simulink model "EDS_Simulink_Model_02"  (R2022a)
settings: Solver=VariableStepAuto  StartTime=0.0  StopTime=stop_time  MaxStep=1e-5  RelTol=1e-3
values from neighbouring files (symbols this model uses):
  a = a/180*pi    [EDS_Script_Model_01.m]    (also in EDS_Script_Model_02.m)
  accel = wheel_radps/accel_time    [EDS_Script_Model_01.m]    (also in EDS_Script_Model_02.m)
  accel_time = 5.33    [EDS_Script_Model_01.m]    (also in EDS_Script_Model_02.m)
  Cx = 0.25    [EDS_Script_Model_01.m]    (also in EDS_Script_Model_02.m)
  d = 1.5    [EDS_Script_Model_01.m]    (also in EDS_Script_Model_02.m)
  density = 1.3    [EDS_Script_Model_01.m]    (also in EDS_Script_Model_02.m)
  F = 4e-04    (= 0.0004)    [EDS_Script_Model_02.m]
  Filter_coefficient = 100/50    (= 2)    [EDS_Script_Model_02.m]
  fr = 0.01    [EDS_Script_Model_01.m]    (also in EDS_Script_Model_02.m)
  g = 9.81    [EDS_Script_Model_01.m]    (also in EDS_Script_Model_02.m)
  i_gear = 7.2    [EDS_Script_Model_01.m]    (also in EDS_Script_Model_02.m = 1)
  J = 0.07/4    (= 0.0175)    [EDS_Script_Model_02.m]
  K_tor_all_1 = 1/2    (= 0.5)    [EDS_Script_Model_01.m]    (also in EDS_Script_Model_02.m)
  K_tor_all_2 = 1/2    (= 0.5)    [EDS_Script_Model_01.m]    (also in EDS_Script_Model_02.m)
  Kd_w = 0.5/8    (= 0.0625)    [EDS_Script_Model_02.m]
  Ki_id = 0.2/14    (= 0.0142857142857)    [EDS_Script_Model_02.m]
  Ki_iq = 10/14    (= 0.714285714286)    [EDS_Script_Model_02.m]
  Ki_w = 2/0.024    (= 83.3333333333)    [EDS_Script_Model_02.m]
  Kp_id = 5/12    (= 0.416666666667)    [EDS_Script_Model_02.m]
  Kp_iq = 30/12    (= 2.5)    [EDS_Script_Model_02.m]
  Kp_w = 55/0.024    (= 2291.66666667)    [EDS_Script_Model_02.m]
  L = 2.5    [EDS_Script_Model_01.m]    (also in EDS_Script_Model_02.m)
  M = 1200    [EDS_Script_Model_01.m]    (also in EDS_Script_Model_02.m)
  n_eff_gear = 0.98    [EDS_Script_Model_01.m]    (also in EDS_Script_Model_02.m = 1)
  p = 4    [EDS_Script_Model_02.m]
  Rs = 4.47-1.47-0.40    (= 2.6)    [EDS_Script_Model_02.m]
  Rw = 0.26    [EDS_Script_Model_01.m]    (also in EDS_Script_Model_02.m)
  S = 1.9    [EDS_Script_Model_01.m]    (also in EDS_Script_Model_02.m)
  Satur_max_PI_id = Vdc_1*sqrt(1/3)    [EDS_Script_Model_02.m]
  Satur_max_PI_iq = Vdc_1*sqrt(1/3)    [EDS_Script_Model_02.m]
  Satur_max_PI_w = 40+30    (= 70)    [EDS_Script_Model_02.m]
  Satur_min_PI_id = -Vdc_1*sqrt(1/3)    [EDS_Script_Model_02.m]
  Satur_min_PI_iq = -Vdc_1*sqrt(1/3)    [EDS_Script_Model_02.m]
  Satur_min_PI_w = -40-30    (= -70)    [EDS_Script_Model_02.m]
  steering_angle_1 = steering_angle_1_m(ii)    [EDS_Script_Model_01.m]    (also in EDS_Script_Model_02.m)
  steering_angle_2 = steering_angle_2_m(ii)    [EDS_Script_Model_01.m]    (also in EDS_Script_Model_02.m)
  steering_angle_3 = steering_angle_3_m(ii)    [EDS_Script_Model_01.m]    (also in EDS_Script_Model_02.m)
  steering_angle_4 = steering_angle_4_m(ii)    [EDS_Script_Model_01.m]    (also in EDS_Script_Model_02.m)
  steering_angle_initial = steering_angle_initial_m(ii)    [EDS_Script_Model_01.m]    (also in EDS_Script_Model_02.m)
  Tf = 0    [EDS_Script_Model_02.m]
  time_steering_angle_1 = 8    [EDS_Script_Model_01.m]    (also in EDS_Script_Model_02.m)
  time_steering_angle_2 = 10    [EDS_Script_Model_01.m]    (also in EDS_Script_Model_02.m)
  time_steering_angle_3 = 14    [EDS_Script_Model_01.m]    (also in EDS_Script_Model_02.m)
  time_steering_angle_4 = 18    [EDS_Script_Model_01.m]    (also in EDS_Script_Model_02.m)
  Vdc_1 = 500    [EDS_Script_Model_02.m]
  Vdc_2 = 500    [EDS_Script_Model_02.m]
  Vf = 0    [EDS_Script_Model_02.m]
  Vfd = 0    [EDS_Script_Model_02.m]
undefined symbols (not defined in the file or in its folder): time_w_ref_1, time_w_ref_2, w_ref_1, w_ref_2, w_ref_initial
libraries: slpidlib x6, spsPermanentMagnetSynchronousMachineLib x2, spsThreePhaseVIMeasurementLib x2, spsUniversalBridgeLib x2, spsDCVoltageSourceLib x2, spsVoltageMeasurementLib x2, spspowerguiLib x1
(part 2 of 2)

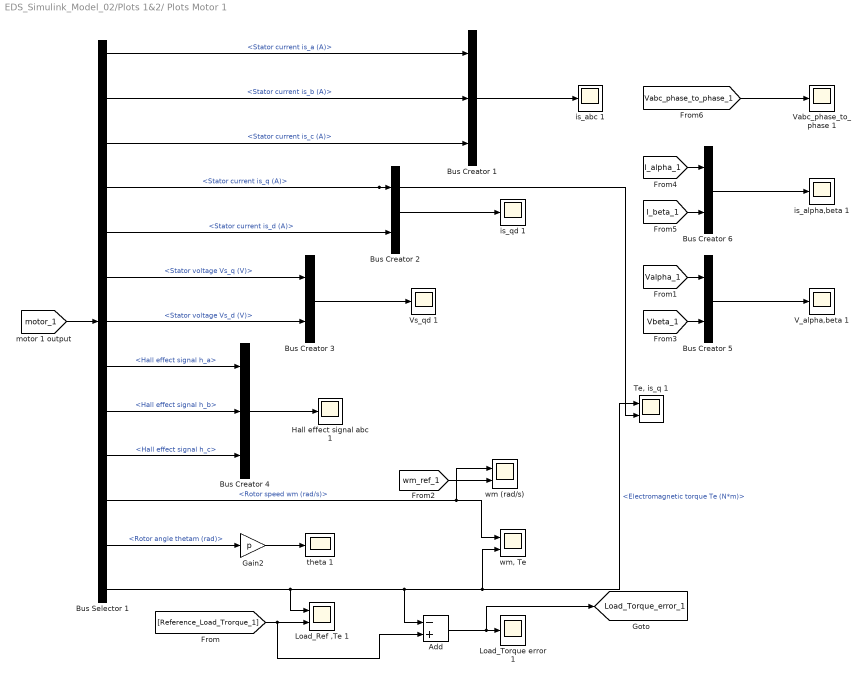
== system EDS_Simulink_Model_02/Plots 1&2/ Plots Motor 1 ==
  Add : Sum  Inputs=-+
  Bus Creator 1 : BusCreator  Inputs=3
  Bus Creator {2..3,5..6} (4 alike) : BusCreator  Inputs=2
  Bus Creator 4 : BusCreator  Inputs=3
  Bus Selector 1 : BusSelector  OutputSignals=Stator current is_a (A),Stator current is_b (A),Stator current is_c (A),Stator current is_q (A),Stator current is_d (A),Stator voltage Vs_q (V),Stator voltage Vs_d (V),Hall effect signal h_a,Hall effect signal h_b,Hall effect signal h_c,Rotor speed wm (rad/s),Rotor angle thetam (rad),Electromagnetic torque Te (N*m)
  Gain2 : Gain  Gain=p
  Hall effect signal abc 1 : Scope
  Load_Ref ,Te 1 : Scope  NumInputPorts=2
  Load_Torque error 1 : Scope
  "Te, is_q 1" : Scope  NumInputPorts=2
  V_alpha,beta 1 : Scope
  Vabc_phase_to_phase 1 : Scope
  Vs_qd 1 : Scope
  is_abc 1 : Scope
  is_alpha,beta 1 : Scope
  is_qd 1 : Scope
  theta 1 : Scope
  wm (rad/s) : Scope  NumInputPorts=2
  "wm, Te" : Scope  NumInputPorts=2
  tag scope: Load_Torque_error_1=global
  wires:
  Bus Creator 2/1 -> is_qd 1/1
  Bus Creator 3/1 -> Vs_qd 1/1
  Bus Creator 4/1 -> Hall effect signal abc 1/1
  Bus Selector 1/7 -> Bus Creator 3/2  "<Stator voltage Vs_d (V)>"
  [Vabc_phase_to_phase_1] -> Vabc_phase_to_phase 1/1
  Bus Selector 1/5 -> Bus Creator 2/2  "<Stator current is_d (A)>"
  Bus Selector 1/3 -> Bus Creator 1/3  "<Stator current is_c (A)>"
  Bus Selector 1/2 -> Bus Creator 1/2  "<Stator current is_b (A)>"
  [Valpha_1] -> Bus Creator 5/1
  [Reference_Load_Trorque_1] -> Add/2, Load_Ref ,Te 1/2
  Bus Selector 1/13 -> "Te, is_q 1"/1, "wm, Te"/2, Add/1, Load_Ref ,Te 1/1  "<Electromagnetic torque Te (N*m)>"
  Bus Selector 1/11 -> wm (rad/s)/1, "wm, Te"/1  "<Rotor speed wm (rad/s)>"
  Bus Selector 1/12 -> Gain2/1  "<Rotor angle thetam (rad)>"
  Bus Creator 5/1 -> V_alpha,beta 1/1
  Bus Selector 1/4 -> "Te, is_q 1"/2, Bus Creator 2/1  "<Stator current is_q (A)>"
  [motor_1] -> Bus Selector 1/1
  Bus Selector 1/10 -> Bus Creator 4/3  "<Hall effect signal h_c>"
  Bus Creator 1/1 -> is_abc 1/1
  Bus Selector 1/6 -> Bus Creator 3/1  "<Stator voltage Vs_q (V)>"
  Bus Selector 1/9 -> Bus Creator 4/2  "<Hall effect signal h_b>"
  [Vbeta_1] -> Bus Creator 5/2
  Bus Selector 1/1 -> Bus Creator 1/1  "<Stator current is_a (A)>"
  [I_alpha_1] -> Bus Creator 6/1
  Bus Selector 1/8 -> Bus Creator 4/1  "<Hall effect signal h_a>"
  [I_beta_1] -> Bus Creator 6/2
  Gain2/1 -> theta 1/1
  Bus Creator 6/1 -> is_alpha,beta 1/1
  Add/1 -> [Load_Torque_error_1], Load_Torque error 1/1
  [wm_ref_1] -> wm (rad/s)/2

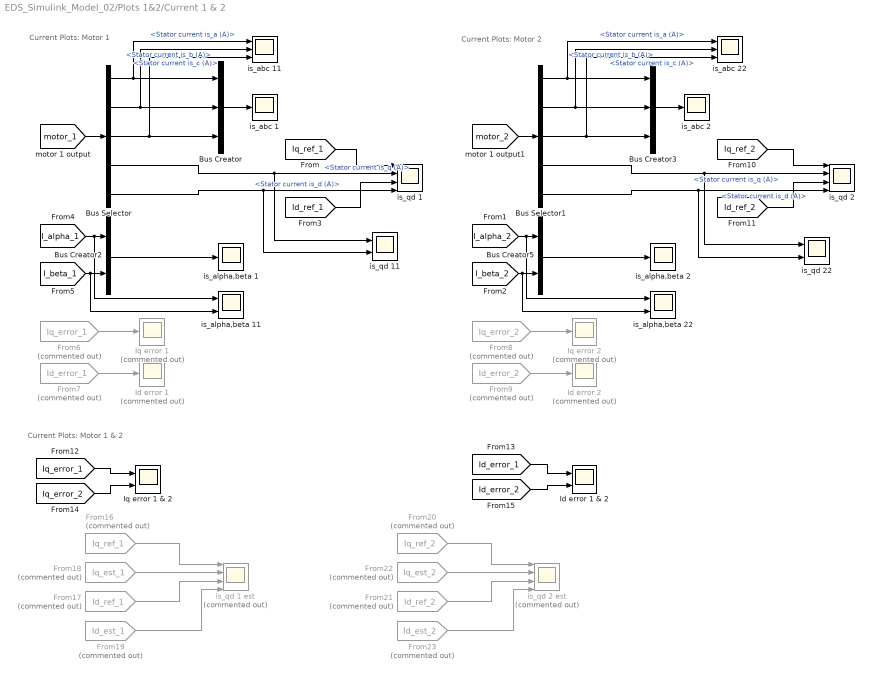
== system EDS_Simulink_Model_02/Plots 1&2/Current 1 & 2 ==
  note: Current Plots: Motor 1 & 2
  note: Current Plots: Motor 1
  note: Current Plots: Motor 2
  Bus Creator : BusCreator  Inputs=3
  Bus Creator2 : BusCreator  Inputs=2
  Bus Creator3 : BusCreator  Inputs=3
  Bus Creator5 : BusCreator  Inputs=2
  Bus Selector : BusSelector  OutputSignals=Stator current is_a (A),Stator current is_b (A),Stator current is_c (A),Stator current is_q (A),Stator current is_d (A)
  Bus Selector1 : BusSelector  OutputSignals=Stator current is_a (A),Stator current is_b (A),Stator current is_c (A),Stator current is_q (A),Stator current is_d (A)
  From16 : From  Commented=on  GotoTag=Iq_ref_1  TagVisibility=global
  From17 : From  Commented=on  GotoTag=Id_ref_1  TagVisibility=global
  From18 : From  Commented=on  GotoTag=Iq_est_1  TagVisibility=global
  From19 : From  Commented=on  GotoTag=Id_est_1  TagVisibility=global
  From20 : From  Commented=on  GotoTag=Iq_ref_2  TagVisibility=global
  From21 : From  Commented=on  GotoTag=Id_ref_2  TagVisibility=global
  From22 : From  Commented=on  GotoTag=Iq_est_2  TagVisibility=global
  From23 : From  Commented=on  GotoTag=Id_est_2  TagVisibility=global
  From6 : From  Commented=on  GotoTag=Iq_error_1  TagVisibility=global
  From7 : From  Commented=on  GotoTag=Id_error_1  TagVisibility=global
  From8 : From  Commented=on  GotoTag=Iq_error_2  TagVisibility=global
  From9 : From  Commented=on  GotoTag=Id_error_2  TagVisibility=global
  Id error 1 : Scope  Commented=on
  Id error 1 & 2 : Scope  NumInputPorts=2
  Id error 2 : Scope  Commented=on
  Iq error 1 : Scope  Commented=on
  Iq error 1 & 2 : Scope  NumInputPorts=2
  Iq error 2 : Scope  Commented=on
  is_abc 1 : Scope
  is_abc 11 : Scope  NumInputPorts=3
  is_abc 2 : Scope
  is_abc 22 : Scope  NumInputPorts=3
  is_alpha,beta 1 : Scope
  is_alpha,beta 11 : Scope  NumInputPorts=2
  is_alpha,beta 2 : Scope
  is_alpha,beta 22 : Scope  NumInputPorts=2
  is_qd 1 : Scope  NumInputPorts=4
  is_qd 1 est : Scope  Commented=on  NumInputPorts=4
  is_qd 11 : Scope  NumInputPorts=2
  is_qd 2 : Scope  NumInputPorts=4
  is_qd 2 est : Scope  Commented=on  NumInputPorts=4
  is_qd 22 : Scope  NumInputPorts=2
  wires:
  From9/1 -> Id error 2/1
  From8/1 -> Iq error 2/1
  [Id_ref_2] -> is_qd 2/3
  [I_alpha_2] -> is_alpha,beta 22/1, Bus Creator5/1
  Bus Selector1/3 -> is_abc 22/3, Bus Creator3/3  "<Stator current is_c (A)>"
  Bus Creator3/1 -> is_abc 2/1
  Bus Creator5/1 -> is_alpha,beta 2/1
  [Iq_ref_2] -> is_qd 2/1
  [motor_2] -> Bus Selector1/1
  From7/1 -> Id error 1/1
  Bus Selector/2 -> is_abc 11/2, Bus Creator/2  "<Stator current is_b (A)>"
  Bus Creator2/1 -> is_alpha,beta 1/1
  Bus Selector/3 -> Bus Creator/3, is_abc 11/3  "<Stator current is_c (A)>"
  From6/1 -> Iq error 1/1
  [Iq_ref_1] -> is_qd 1/1
  [Id_ref_1] -> is_qd 1/3
  Bus Selector/5 -> is_qd 11/2, is_qd 1/4  "<Stator current is_d (A)>"
  Bus Creator/1 -> is_abc 1/1
  [I_alpha_1] -> is_alpha,beta 11/1, Bus Creator2/1
  [motor_1] -> Bus Selector/1
  [I_beta_1] -> Bus Creator2/2, is_alpha,beta 11/2
  Bus Selector/4 -> is_qd 11/1, is_qd 1/2  "<Stator current is_q (A)>"
  Bus Selector/1 -> is_abc 11/1, Bus Creator/1  "<Stator current is_a (A)>"
  [Id_error_2] -> Id error 1 & 2/2
  [Iq_error_2] -> Iq error 1 & 2/2
  [Id_error_1] -> Id error 1 & 2/1
  [Iq_error_1] -> Iq error 1 & 2/1
  From16/1 -> is_qd 1 est/1
  From18/1 -> is_qd 1 est/2
  From17/1 -> is_qd 1 est/3
  From19/1 -> is_qd 1 est/4
  From21/1 -> is_qd 2 est/3
  From20/1 -> is_qd 2 est/1
  From22/1 -> is_qd 2 est/2
  From23/1 -> is_qd 2 est/4
  Bus Selector1/4 -> is_qd 22/1, is_qd 2/2  "<Stator current is_q (A)>"
  Bus Selector1/5 -> is_qd 22/2, is_qd 2/4  "<Stator current is_d (A)>"
  Bus Selector1/2 -> is_abc 22/2, Bus Creator3/2  "<Stator current is_b (A)>"
  Bus Selector1/1 -> is_abc 22/1, Bus Creator3/1  "<Stator current is_a (A)>"
  [I_beta_2] -> is_alpha,beta 22/2, Bus Creator5/2

== system EDS_Simulink_Model_02/Plots 1&2/EDS ==
  Difference Speed Δω : Scope
  Speed ωref & ωv : Scope  NumInputPorts=2
  Steering Angle δ : Scope
  wires:
  [Reference_Speed] -> Speed ωref & ωv/2
  [Center_of_turn_Angular_Speed] -> Speed ωref & ωv/1
  [Steering_Angle] -> Steering Angle δ/1
  [Difference_Speed] -> Difference Speed Δω/1

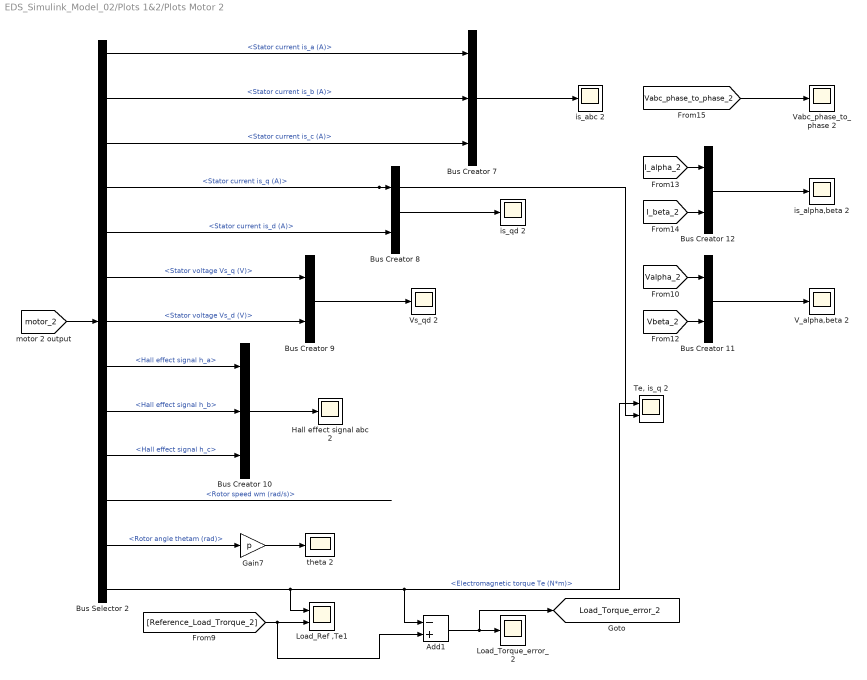
== system EDS_Simulink_Model_02/Plots 1&2/Plots Motor 2 ==
  Add1 : Sum  Inputs=-+
  Bus Creator 10 : BusCreator  Inputs=3
  Bus Creator {8..9,11..12} (4 alike) : BusCreator  Inputs=2
  Bus Creator 7 : BusCreator  Inputs=3
  Bus Selector 2 : BusSelector  OutputSignals=Stator current is_a (A),Stator current is_b (A),Stator current is_c (A),Stator current is_q (A),Stator current is_d (A),Stator voltage Vs_q (V),Stator voltage Vs_d (V),Hall effect signal h_a,Hall effect signal h_b,Hall effect signal h_c,Rotor speed wm (rad/s),Rotor angle thetam (rad),Electromagnetic torque Te (N*m)
  Gain7 : Gain  Gain=p
  Hall effect signal abc 2 : Scope
  Load_Ref ,Te1 : Scope  NumInputPorts=2
  Load_Torque_error_2 : Scope
  "Te, is_q 2" : Scope  NumInputPorts=2
  V_alpha,beta 2 : Scope
  Vabc_phase_to_phase 2 : Scope
  Vs_qd 2 : Scope
  is_abc 2 : Scope
  is_alpha,beta 2 : Scope
  is_qd 2 : Scope
  theta 2 : Scope
  tag scope: Load_Torque_error_2=global
  wires:
  Add1/1 -> [Load_Torque_error_2], Load_Torque_error_2/1
  Bus Selector 2/12 -> Gain7/1  "<Rotor angle thetam (rad)>"
  Bus Selector 2/7 -> Bus Creator 9/2  "<Stator voltage Vs_d (V)>"
  Bus Selector 2/2 -> Bus Creator 7/2  "<Stator current is_b (A)>"
  Bus Creator 8/1 -> is_qd 2/1
  Bus Creator 10/1 -> Hall effect signal abc 2/1
  [Reference_Load_Trorque_2] -> Add1/2, Load_Ref ,Te1/2
  Gain7/1 -> theta 2/1
  [Vabc_phase_to_phase_2] -> Vabc_phase_to_phase 2/1
  Bus Selector 2/9 -> Bus Creator 10/2  "<Hall effect signal h_b>"
  Bus Selector 2/4 -> "Te, is_q 2"/2, Bus Creator 8/1  "<Stator current is_q (A)>"
  Bus Creator 7/1 -> is_abc 2/1
  Bus Selector 2/10 -> Bus Creator 10/3  "<Hall effect signal h_c>"
  Bus Selector 2/8 -> Bus Creator 10/1  "<Hall effect signal h_a>"
  Bus Selector 2/6 -> Bus Creator 9/1  "<Stator voltage Vs_q (V)>"
  Bus Creator 12/1 -> is_alpha,beta 2/1
  Bus Selector 2/13 -> "Te, is_q 2"/1, Add1/1, Load_Ref ,Te1/1  "<Electromagnetic torque Te (N*m)>"
  [motor_2] -> Bus Selector 2/1
  [Valpha_2] -> Bus Creator 11/1
  Bus Creator 11/1 -> V_alpha,beta 2/1
  Bus Selector 2/3 -> Bus Creator 7/3  "<Stator current is_c (A)>"
  [I_beta_2] -> Bus Creator 12/2
  [Vbeta_2] -> Bus Creator 11/2
  Bus Selector 2/1 -> Bus Creator 7/1  "<Stator current is_a (A)>"
  Bus Selector 2/5 -> Bus Creator 8/2  "<Stator current is_d (A)>"
  [I_alpha_2] -> Bus Creator 12/1
  Bus Creator 9/1 -> Vs_qd 2/1
  Bus Selector 2/11 -> ?  "<Rotor speed wm (rad/s)>"

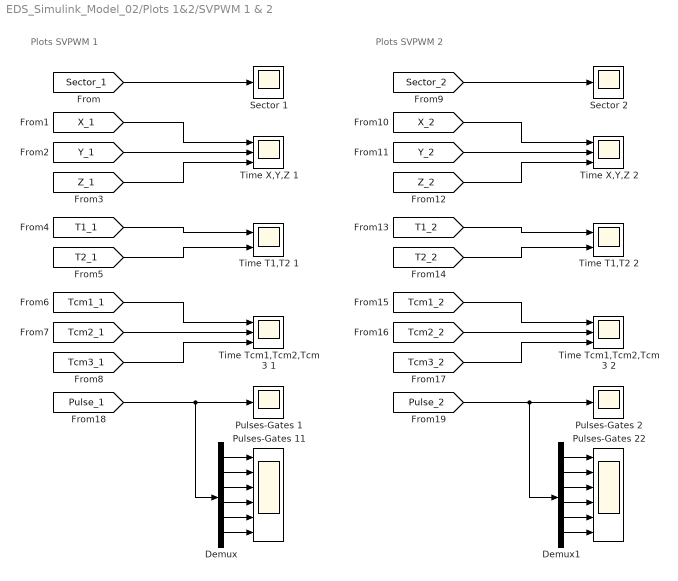
== system EDS_Simulink_Model_02/Plots 1&2/SVPWM 1 & 2 ==
  note: Plots SVPWM 2
  note: Plots SVPWM 1
  Demux : Demux  Outputs=6
  Demux1 : Demux  Outputs=6
  Pulses-Gates 1 : Scope
  Pulses-Gates 11 : Scope  NumInputPorts=6
  Pulses-Gates 2 : Scope
  Pulses-Gates 22 : Scope  NumInputPorts=6
  Sector 1 : Scope
  Sector 2 : Scope
  Time T1,T2 1 : Scope  NumInputPorts=2
  Time T1,T2 2 : Scope  NumInputPorts=2
  Time Tcm1,Tcm2,Tcm3 1 : Scope  NumInputPorts=3
  Time Tcm1,Tcm2,Tcm3 2 : Scope  NumInputPorts=3
  Time X,Y,Z 1 : Scope  NumInputPorts=3
  Time X,Y,Z 2 : Scope  NumInputPorts=3
  wires:
  [Tcm1_1] -> Time Tcm1,Tcm2,Tcm3 1/1
  [X_1] -> Time X,Y,Z 1/1
  [Tcm3_1] -> Time Tcm1,Tcm2,Tcm3 1/3
  [Pulse_1] -> Pulses-Gates 1/1, Demux/1
  [T2_1] -> Time T1,T2 1/2
  [T1_1] -> Time T1,T2 1/1
  [Z_1] -> Time X,Y,Z 1/3
  [Sector_1] -> Sector 1/1
  [Y_1] -> Time X,Y,Z 1/2
  [Tcm2_1] -> Time Tcm1,Tcm2,Tcm3 1/2
  [Tcm3_2] -> Time Tcm1,Tcm2,Tcm3 2/3
  [Y_2] -> Time X,Y,Z 2/2
  [T2_2] -> Time T1,T2 2/2
  [Sector_2] -> Sector 2/1
  [Tcm1_2] -> Time Tcm1,Tcm2,Tcm3 2/1
  [T1_2] -> Time T1,T2 2/1
  [X_2] -> Time X,Y,Z 2/1
  [Pulse_2] -> Demux1/1, Pulses-Gates 2/1
  [Z_2] -> Time X,Y,Z 2/3
  [Tcm2_2] -> Time Tcm1,Tcm2,Tcm3 2/2
  Demux/1 -> Pulses-Gates 11/1
  Demux/2 -> Pulses-Gates 11/2
  Demux/3 -> Pulses-Gates 11/3
  Demux/4 -> Pulses-Gates 11/4
  Demux/5 -> Pulses-Gates 11/5
  Demux/6 -> Pulses-Gates 11/6
  Demux1/5 -> Pulses-Gates 22/5
  Demux1/2 -> Pulses-Gates 22/2
  Demux1/3 -> Pulses-Gates 22/3
  Demux1/1 -> Pulses-Gates 22/1
  Demux1/4 -> Pulses-Gates 22/4
  Demux1/6 -> Pulses-Gates 22/6

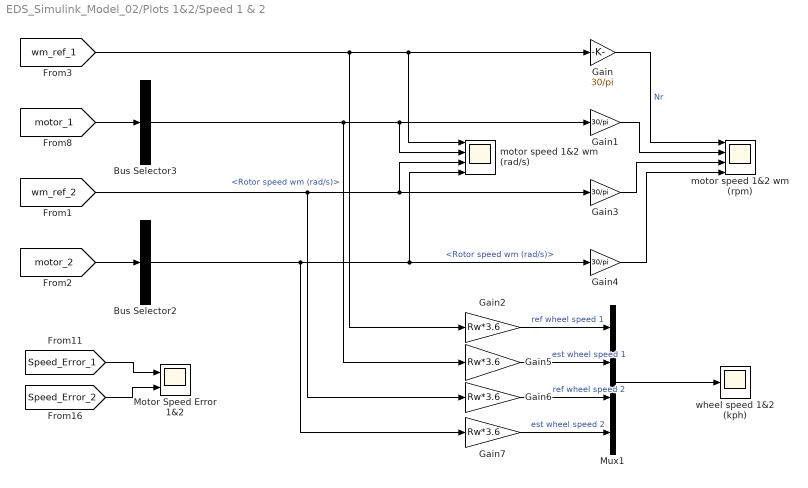
== system EDS_Simulink_Model_02/Plots 1&2/Speed 1 & 2 ==
  Bus Selector2 : BusSelector  OutputSignals=Rotor speed wm (rad/s)
  Bus Selector3 : BusSelector  OutputSignals=Rotor speed wm (rad/s)
  Gain{,1,3..4} (4 alike) : Gain  Gain=30/pi
  Gain{2,5..7} (4 alike) : Gain  Gain=Rw*3.6
  Motor Speed Error 1&2 : Scope  NumInputPorts=2
  Mux1 : Mux
  motor speed 1&2 wm (rad/s) : Scope  NumInputPorts=4
  motor speed 1&2 wm (rpm) : Scope  NumInputPorts=4
  wheel speed 1&2 (kph) : Scope
  wires:
  [wm_ref_2] -> Gain6/1, Gain3/1, motor speed 1&2 wm (rad/s)/3
  [motor_2] -> Bus Selector2/1
  Bus Selector2/1 -> Gain7/1, Gain4/1, motor speed 1&2 wm (rad/s)/4  "<Rotor speed wm (rad/s)>"
  Bus Selector3/1 -> Gain5/1, Gain1/1, motor speed 1&2 wm (rad/s)/2  "<Rotor speed wm (rad/s)>"
  [wm_ref_1] -> Gain2/1, Gain/1, motor speed 1&2 wm (rad/s)/1
  Gain/1 -> motor speed 1&2 wm (rpm)/1  "Nr"
  Gain1/1 -> motor speed 1&2 wm (rpm)/2
  Gain3/1 -> motor speed 1&2 wm (rpm)/3
  Gain4/1 -> motor speed 1&2 wm (rpm)/4
  Gain7/1 -> Mux1/4  "est wheel speed 2"
  Gain6/1 -> Mux1/3  "ref wheel speed 2"
  Gain5/1 -> Mux1/2  "est wheel speed 1"
  Gain2/1 -> Mux1/1  "ref wheel speed 1"
  Mux1/1 -> wheel speed 1&2 (kph)/1
  [Speed_Error_2] -> Motor Speed Error 1&2/2
  [Speed_Error_1] -> Motor Speed Error 1&2/1
  [motor_1] -> Bus Selector3/1

== system EDS_Simulink_Model_02/Plots 1&2/Torque 1 & 2 ==
  Add : Sum  Inputs=-+
  Add1 : Sum  Inputs=-+
  Bus Selector : BusSelector  OutputSignals=Electromagnetic torque Te (N*m)
  Bus Selector1 : BusSelector  OutputSignals=Electromagnetic torque Te (N*m)
  Electrical Motor Torque 1 & 2 : Scope  NumInputPorts=2
  Goto : Goto  Commented=on  GotoTag=Load_Torque_error_1  TagVisibility=global
  Goto1 : Goto  Commented=on  GotoTag=Load_Torque_error_1  TagVisibility=global
  Load Torque error 1 & 2 : Scope  NumInputPorts=2
  Load Wheel Torque 1 & 2 : Scope  NumInputPorts=4
  Wheel Torque 1 & 2 : Scope  NumInputPorts=4
  wires:
  Add/1 -> Goto/1, Load Torque error 1 & 2/1
  Add1/1 -> Load Torque error 1 & 2/2, Goto1/1
  [Load_Wheel_Torque_2] -> Wheel Torque 1 & 2/4, Add1/2
  [Load_Wheel_Torque_1] -> Add/2, Wheel Torque 1 & 2/2  "est"
  Bus Selector1/1 -> Electrical Motor Torque 1 & 2/2, Wheel Torque 1 & 2/3, Add1/1  "<Electromagnetic torque Te (N*m)>"
  Bus Selector/1 -> Electrical Motor Torque 1 & 2/1, Add/1, Wheel Torque 1 & 2/1  "<Electromagnetic torque Te (N*m)>"
  [motor_2] -> Bus Selector1/1
  [motor_1] -> Bus Selector/1
  [Ref_Load_Wheel_Torque_1] -> Load Wheel Torque 1 & 2/1
  [Load_Wheel_Torque_1] -> Load Wheel Torque 1 & 2/2
  [Ref_Load_Motor_Torque_2] -> Load Wheel Torque 1 & 2/3
  [Load_Wheel_Torque_2] -> Load Wheel Torque 1 & 2/4

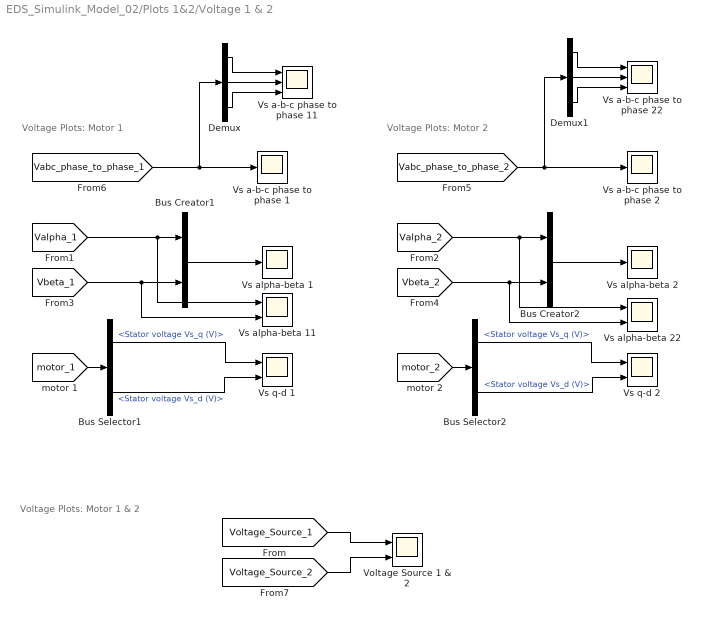
== system EDS_Simulink_Model_02/Plots 1&2/Voltage 1 & 2 ==
  note: Voltage Plots: Motor 1 & 2
  note: Voltage Plots: Motor 2
  note: Voltage Plots: Motor 1
  Bus Creator1 : BusCreator  Inputs=2
  Bus Creator2 : BusCreator  Inputs=2
  Bus Selector1 : BusSelector  OutputSignals=Stator voltage Vs_q (V),Stator voltage Vs_d (V)
  Bus Selector2 : BusSelector  OutputSignals=Stator voltage Vs_q (V),Stator voltage Vs_d (V)
  Demux : Demux  Outputs=3
  Demux1 : Demux  Outputs=3
  Voltage Source 1 & 2 : Scope  NumInputPorts=2
  Vs a-b-c phase to phase 1 : Scope
  Vs a-b-c phase to phase 11 : Scope  NumInputPorts=3
  Vs a-b-c phase to phase 2 : Scope
  Vs a-b-c phase to phase 22 : Scope  NumInputPorts=3
  Vs alpha-beta 1 : Scope
  Vs alpha-beta 11 : Scope  NumInputPorts=2
  Vs alpha-beta 2 : Scope
  Vs alpha-beta 22 : Scope  NumInputPorts=2
  Vs q-d 1 : Scope  NumInputPorts=2
  Vs q-d 2 : Scope  NumInputPorts=2
  wires:
  [motor_1] -> Bus Selector1/1
  [Valpha_1] -> Vs alpha-beta 11/1, Bus Creator1/1
  Bus Creator1/1 -> Vs alpha-beta 1/1
  Bus Selector1/1 -> Vs q-d 1/1  "<Stator voltage Vs_q (V)>"
  Bus Selector1/2 -> Vs q-d 1/2  "<Stator voltage Vs_d (V)>"
  [Vbeta_1] -> Vs alpha-beta 11/2, Bus Creator1/2
  [Vabc_phase_to_phase_1] -> Vs a-b-c phase to phase 1/1, Demux/1
  [motor_2] -> Bus Selector2/1
  Bus Selector2/1 -> Vs q-d 2/1  "<Stator voltage Vs_q (V)>"
  Bus Creator2/1 -> Vs alpha-beta 2/1
  [Valpha_2] -> Vs alpha-beta 22/1, Bus Creator2/1
  Bus Selector2/2 -> Vs q-d 2/2  "<Stator voltage Vs_d (V)>"
  [Vbeta_2] -> Vs alpha-beta 22/2, Bus Creator2/2
  [Voltage_Source_2] -> Voltage Source 1 & 2/2
  [Voltage_Source_1] -> Voltage Source 1 & 2/1
  Demux/1 -> Vs a-b-c phase to phase 11/1
  Demux/2 -> Vs a-b-c phase to phase 11/2
  Demux/3 -> Vs a-b-c phase to phase 11/3
  Demux1/3 -> Vs a-b-c phase to phase 22/3
  Demux1/2 -> Vs a-b-c phase to phase 22/2
  Demux1/1 -> Vs a-b-c phase to phase 22/1
  [Vabc_phase_to_phase_2] -> Demux1/1, Vs a-b-c phase to phase 2/1

== system EDS_Simulink_Model_02/Control Systetm 1 (FOC & SVPWM)/SVPWM 1/Calculation of Action Time T1,T2 1 ==
  note: z
  note: y
  note: -z
  note: -x
  note: x
  note: -y
  note: y
  note: -x
  note: x
  note: z
  note: -y
  note: -z
  note: T1
  note: T2
  note: T
  note: T1
  note: T2
  N : Inport
  X : Inport  Port=2
  Y : Inport  Port=3
  Z : Inport  Port=4
  T : Inport  Port=5
  " " : Gain  Gain=-1
  "  " : Gain  Gain=-1
  "    " : Gain  Gain=-1
  Fcn : Fcn  Expr=u(3)-u(2)-u(1)
  Fcn1 : Fcn  Expr=u(1)*u(3)/(u(1)+u(2))
  Fcn2 : Fcn  Expr=u(2)*u(3)/(u(1)+u(2))
  Multiport Switch : MultiPortSwitch  Inputs=6  DiagnosticForDefault=None  SaturateOnIntegerOverflow=off  InputSameDT=off
  Multiport Switch1 : MultiPortSwitch  Inputs=6  DiagnosticForDefault=None  SaturateOnIntegerOverflow=off  InputSameDT=off
  Mux : Mux  Inputs=3
  Switch : Switch  SaturateOnIntegerOverflow=off  InputSameDT=off
  Switch1 : Switch  Criteria=u2 > Threshold  SaturateOnIntegerOverflow=off  InputSameDT=off
  T1 : Outport  VectorParamsAs1DForOutWhenUnconnected=off
  T2 : Outport  Port=2  VectorParamsAs1DForOutWhenUnconnected=off
  wires:
  N/1 -> Multiport Switch1/1, Multiport Switch/1
  X/1 -> Multiport Switch1/4, Multiport Switch/6, " "/1
  Y/1 -> Multiport Switch1/2, Multiport Switch/3, "  "/1
  Z/1 -> Multiport Switch1/5, Multiport Switch/2, "    "/1
  "    "/1 -> Multiport Switch1/7, Multiport Switch/4
  "  "/1 -> Multiport Switch/7, Multiport Switch1/6
  " "/1 -> Multiport Switch/5, Multiport Switch1/3
  Multiport Switch/1 -> Mux/1, Switch/1
  Multiport Switch1/1 -> Switch1/1, Mux/2
  T/1 -> Mux/3
  Mux/1 -> Fcn/1, Fcn1/1, Fcn2/1
  Fcn/1 -> Switch/2, Switch1/2
  Fcn1/1 -> Switch/3
  Fcn2/1 -> Switch1/3
  Switch/1 -> T1/1
  Switch1/1 -> T2/1

== system EDS_Simulink_Model_02/Control Systetm 1 (FOC & SVPWM)/SVPWM 1/Calculation of X,Y,Z 1 ==
  T : Inport
  Valpha : Inport  Port=2
  Vbeta : Inport  Port=3
  Vdc : Inport  Port=4
  Divide : Product  Inputs=**/
  Divide1 : Product  Inputs=**/
  Divide2 : Product  Inputs=**/
  Gain : Gain  Gain=sqrt(3)/3
  Gain1 : Gain  Gain=sqrt(3)
  Gain2 : Gain  Gain=1.5
  Gain3 : Gain  Gain=1.5
  Subtract : Sum
  Subtract1 : Sum  Inputs=+-
  X : Outport  VectorParamsAs1DForOutWhenUnconnected=off
  Y : Outport  Port=2  VectorParamsAs1DForOutWhenUnconnected=off
  Z : Outport  Port=3  VectorParamsAs1DForOutWhenUnconnected=off
  wires:
  Gain/1 -> Subtract1/1, Subtract/1
  Gain1/1 -> Divide/1
  T/1 -> Divide2/2, Divide1/2, Divide/2
  Vdc/1 -> Divide2/3, Divide1/3, Divide/3
  Valpha/1 -> Subtract1/2, Subtract/2
  Subtract/1 -> Divide1/1
  Subtract1/1 -> Divide2/1
  Divide/1 -> X/1
  Divide1/1 -> Gain2/1
  Divide2/1 -> Gain3/1
  Gain2/1 -> Y/1
  Gain3/1 -> Z/1
  Vbeta/1 -> Gain/1, Gain1/1

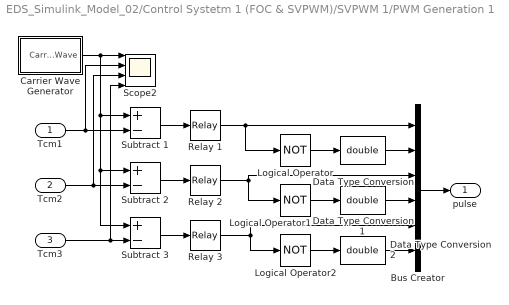
== system EDS_Simulink_Model_02/Control Systetm 1 (FOC & SVPWM)/SVPWM 1/PWM Generation 1 ==
  Tcm1 : Inport
  Tcm2 : Inport  Port=2
  Tcm3 : Inport  Port=3
  Bus Creator : BusCreator  Inputs=6
  Carrier Wave Generator : Subsystem
  Data Type Conversion : DataTypeConversion  OutDataTypeStr=double  SaturateOnIntegerOverflow=off  RndMeth=Floor
  Data Type Conversion1 : DataTypeConversion  OutDataTypeStr=double  SaturateOnIntegerOverflow=off  RndMeth=Floor
  Data Type Conversion2 : DataTypeConversion  OutDataTypeStr=double  SaturateOnIntegerOverflow=off  RndMeth=Floor
  Logical Operator1 : Logic  Operator=NOT  AllPortsSameDT=off
  Logical Operator2 : Logic  Operator=NOT  AllPortsSameDT=off
  Logical Operator : Logic  Operator=NOT  AllPortsSameDT=off
  Relay 1 : Relay
  Relay 2 : Relay
  Relay 3 : Relay
  Scope2 : Scope  NumInputPorts=4
  Subtract 1 : Sum  Inputs=+-
  Subtract 2 : Sum  Inputs=+-
  Subtract 3 : Sum  Inputs=+-
  pulse : Outport  VectorParamsAs1DForOutWhenUnconnected=off
  wires:
  Subtract 1/1 -> Relay 1/1
  Subtract 2/1 -> Relay 2/1
  Subtract 3/1 -> Relay 3/1
  Logical Operator1/1 -> Data Type Conversion1/1
  Logical Operator2/1 -> Data Type Conversion2/1
  Logical Operator/1 -> Data Type Conversion/1
  Relay 1/1 -> Bus Creator/1, Logical Operator/1
  Relay 2/1 -> Bus Creator/3, Logical Operator1/1
  Relay 3/1 -> Bus Creator/5, Logical Operator2/1
  Bus Creator/1 -> pulse/1
  Data Type Conversion/1 -> Bus Creator/2
  Data Type Conversion1/1 -> Bus Creator/4
  Data Type Conversion2/1 -> Bus Creator/6
  Tcm1/1 -> Scope2/2, Subtract 1/2
  Carrier Wave Generator/1(Carrier Wave) -> Subtract 3/1, Subtract 2/1, Subtract 1/1, Scope2/1
  Tcm3/1 -> Scope2/4, Subtract 3/2
  Tcm2/1 -> Scope2/3, Subtract 2/2

== system EDS_Simulink_Model_02/Control Systetm 1 (FOC & SVPWM)/SVPWM 1/Sector Identification 1 ==
  Valpha : Inport
  Vbeta : Inport  Port=2
  Constant : Constant
  Constant1 : Constant  Value=0
  Gain : Gain  Gain=1.732
  Gain1 : Gain  Gain=-1.732
  Gain2 : Gain  Gain=2
  Gain3 : Gain  Gain=4
  Sum : Sum  Inputs=|-+
  Sum1 : Sum  Inputs=|-+
  Sum2 : Sum  Inputs=|+++
  Switch 1 : Switch  SaturateOnIntegerOverflow=off  InputSameDT=off
  Switch 2 : Switch  SaturateOnIntegerOverflow=off  InputSameDT=off
  Switch 3 : Switch  SaturateOnIntegerOverflow=off  InputSameDT=off
  N : Outport  VectorParamsAs1DForOutWhenUnconnected=off
  wires:
  Vbeta/1 -> Switch 1/2, Sum/1, Sum1/1
  Constant/1 -> Switch 1/1, Switch 3/1, Switch 2/1
  Valpha/1 -> Gain1/1, Gain/1
  Gain/1 -> Sum/2
  Sum/1 -> Switch 2/2
  Sum1/1 -> Switch 3/2
  Gain1/1 -> Sum1/2
  Constant1/1 -> Switch 1/3, Switch 2/3, Switch 3/3
  Switch 2/1 -> Gain2/1
  Switch 3/1 -> Gain3/1
  Gain2/1 -> Sum2/2
  Switch 1/1 -> Sum2/1
  Gain3/1 -> Sum2/3
  Sum2/1 -> N/1  "Sector"

== system EDS_Simulink_Model_02/Control Systetm 1 (FOC & SVPWM)/SVPWM 1/Three Phase Time Comparison Generation 1 ==
  note: Ta
  note: Tb
  note: Tc
  note: b
  note: a
  note: a
  note: c
  note: c
  note: b
  note: a
  note: c
  note: b
  note: b
  note: a
  note: c
  note: c
  note: b
  note: c
  note: a
  note: b
  note: a
  T1 : Inport
  T2 : Inport  Port=2
  T : Inport  Port=3
  N : Inport  Port=4
  Gain1 : Gain  Gain=1/4
  Gain2 : Gain  Gain=1/2
  Gain3 : Gain  Gain=1/2
  Multiport Switch : MultiPortSwitch  Inputs=6  DiagnosticForDefault=None  SaturateOnIntegerOverflow=off  InputSameDT=off
  Multiport Switch1 : MultiPortSwitch  Inputs=6  DiagnosticForDefault=None  SaturateOnIntegerOverflow=off  InputSameDT=off
  Multiport Switch2 : MultiPortSwitch  Inputs=6  DiagnosticForDefault=None  SaturateOnIntegerOverflow=off  InputSameDT=off
  Subtract1 : Sum  Inputs=--+
  Subtract2 : Sum
  Subtract3 : Sum
  Tcm1 : Outport  VectorParamsAs1DForOutWhenUnconnected=off
  Tcm2 : Outport  Port=2  VectorParamsAs1DForOutWhenUnconnected=off
  Tcm3 : Outport  Port=3  VectorParamsAs1DForOutWhenUnconnected=off
  wires:
  T2/1 -> Gain2/1, Subtract1/2
  T/1 -> Subtract1/3
  T1/1 -> Gain3/1, Subtract1/1
  Gain3/1 -> Subtract2/1
  Subtract1/1 -> Gain1/1
  Gain1/1 -> Subtract2/2, Multiport Switch2/5, Multiport Switch2/7, Multiport Switch/3, Multiport Switch/4, Multiport Switch1/2, Multiport Switch1/6
  Subtract2/1 -> Subtract3/2, Multiport Switch/2, Multiport Switch/7, Multiport Switch1/4, Multiport Switch1/5, Multiport Switch2/3, Multiport Switch2/6
  Gain2/1 -> Subtract3/1
  N/1 -> Multiport Switch/1, Multiport Switch2/1, Multiport Switch1/1
  Multiport Switch/1 -> Tcm1/1
  Multiport Switch1/1 -> Tcm2/1
  Multiport Switch2/1 -> Tcm3/1
  Subtract3/1 -> Multiport Switch/5, Multiport Switch/6, Multiport Switch1/3, Multiport Switch1/7, Multiport Switch2/2, Multiport Switch2/4

== system EDS_Simulink_Model_02/Control Systetm 2 (FOC & SVPWM)/SVPWM 2/N2 ==
  Valpha : Inport
  Vbeta : Inport  Port=2
  Constant : Constant
  Constant1 : Constant  Value=0
  Gain : Gain  Gain=1.732
  Gain1 : Gain  Gain=-1.732
  Gain2 : Gain  Gain=2
  Gain3 : Gain  Gain=4
  Sum : Sum  Inputs=|-+
  Sum1 : Sum  Inputs=|-+
  Sum2 : Sum  Inputs=|+++
  Switch : Switch  SaturateOnIntegerOverflow=off  InputSameDT=off
  Switch1 : Switch  SaturateOnIntegerOverflow=off  InputSameDT=off
  Switch2 : Switch  SaturateOnIntegerOverflow=off  InputSameDT=off
  N : Outport  VectorParamsAs1DForOutWhenUnconnected=off
  wires:
  Vbeta/1 -> Switch/2, Sum/1, Sum1/1
  Constant/1 -> Switch/1, Switch2/1, Switch1/1
  Valpha/1 -> Gain1/1, Gain/1
  Gain/1 -> Sum/2
  Sum/1 -> Switch1/2
  Sum1/1 -> Switch2/2
  Gain1/1 -> Sum1/2
  Constant1/1 -> Switch/3, Switch1/3, Switch2/3
  Switch1/1 -> Gain2/1
  Switch2/1 -> Gain3/1
  Gain2/1 -> Sum2/2
  Switch/1 -> Sum2/1
  Gain3/1 -> Sum2/3
  Sum2/1 -> N/1

== system EDS_Simulink_Model_02/Control Systetm 2 (FOC & SVPWM)/SVPWM 2/Subsystem ==
  note: z
  note: y
  note: -z
  note: -x
  note: x
  note: -y
  note: y
  note: -x
  note: x
  note: z
  note: -y
  note: -z
  note: T1
  note: T2
  note: T
  note: T1
  note: T2
  N : Inport
  X : Inport  Port=2
  Y : Inport  Port=3
  Z : Inport  Port=4
  T : Inport  Port=5
  " " : Gain  Gain=-1
  "  " : Gain  Gain=-1
  "    " : Gain  Gain=-1
  Fcn : Fcn  Expr=u(3)-u(2)-u(1)
  Fcn1 : Fcn  Expr=u(1)*u(3)/(u(1)+u(2))
  Fcn2 : Fcn  Expr=u(2)*u(3)/(u(1)+u(2))
  Multiport Switch : MultiPortSwitch  Inputs=6  DiagnosticForDefault=None  SaturateOnIntegerOverflow=off  InputSameDT=off
  Multiport Switch1 : MultiPortSwitch  Inputs=6  DiagnosticForDefault=None  SaturateOnIntegerOverflow=off  InputSameDT=off
  Mux : Mux  Inputs=3
  Switch : Switch  SaturateOnIntegerOverflow=off  InputSameDT=off
  Switch1 : Switch  Criteria=u2 > Threshold  SaturateOnIntegerOverflow=off  InputSameDT=off
  T1 : Outport  VectorParamsAs1DForOutWhenUnconnected=off
  T2 : Outport  Port=2  VectorParamsAs1DForOutWhenUnconnected=off
  wires:
  N/1 -> Multiport Switch1/1, Multiport Switch/1
  X/1 -> Multiport Switch1/4, Multiport Switch/6, " "/1
  Y/1 -> Multiport Switch1/2, Multiport Switch/3, "  "/1
  Z/1 -> Multiport Switch1/5, Multiport Switch/2, "    "/1
  "    "/1 -> Multiport Switch1/7, Multiport Switch/4
  "  "/1 -> Multiport Switch/7, Multiport Switch1/6
  " "/1 -> Multiport Switch/5, Multiport Switch1/3
  Multiport Switch/1 -> Mux/1, Switch/1
  Multiport Switch1/1 -> Switch1/1, Mux/2
  T/1 -> Mux/3
  Mux/1 -> Fcn/1, Fcn1/1, Fcn2/1
  Fcn/1 -> Switch/2, Switch1/2
  Fcn1/1 -> Switch/3
  Fcn2/1 -> Switch1/3
  Switch/1 -> T1/1
  Switch1/1 -> T2/1

== system EDS_Simulink_Model_02/Control Systetm 2 (FOC & SVPWM)/SVPWM 2/Subsystem1 ==
  note: Ta
  note: Tb
  note: Tc
  note: b
  note: a
  note: a
  note: c
  note: c
  note: b
  note: a
  note: c
  note: b
  note: b
  note: a
  note: c
  note: c
  note: b
  note: c
  note: a
  note: b
  note: a
  T1 : Inport
  T2 : Inport  Port=2
  T : Inport  Port=3
  N : Inport  Port=4
  Gain1 : Gain  Gain=1/4
  Gain2 : Gain  Gain=0.5
  Gain3 : Gain  Gain=0.5
  Multiport Switch : MultiPortSwitch  Inputs=6  DiagnosticForDefault=None  SaturateOnIntegerOverflow=off  InputSameDT=off
  Multiport Switch1 : MultiPortSwitch  Inputs=6  DiagnosticForDefault=None  SaturateOnIntegerOverflow=off  InputSameDT=off
  Multiport Switch2 : MultiPortSwitch  Inputs=6  DiagnosticForDefault=None  SaturateOnIntegerOverflow=off  InputSameDT=off
  Subtract1 : Sum  Inputs=--+
  Subtract2 : Sum
  Subtract3 : Sum
  Tcm1 : Outport  VectorParamsAs1DForOutWhenUnconnected=off
  Tcm2 : Outport  Port=2  VectorParamsAs1DForOutWhenUnconnected=off
  Tcm3 : Outport  Port=3  VectorParamsAs1DForOutWhenUnconnected=off
  wires:
  T2/1 -> Gain2/1, Subtract1/2
  T/1 -> Subtract1/3
  T1/1 -> Gain3/1, Subtract1/1
  Gain3/1 -> Subtract2/1
  Subtract1/1 -> Gain1/1
  Gain1/1 -> Subtract2/2, Multiport Switch/3, Multiport Switch/4, Multiport Switch1/2, Multiport Switch1/6, Multiport Switch2/5, Multiport Switch2/7
  Subtract2/1 -> Subtract3/2, Multiport Switch/2, Multiport Switch/7, Multiport Switch1/4, Multiport Switch1/5, Multiport Switch2/3, Multiport Switch2/6
  Gain2/1 -> Subtract3/1
  N/1 -> Multiport Switch/1, Multiport Switch2/1, Multiport Switch1/1
  Multiport Switch/1 -> Tcm1/1
  Multiport Switch1/1 -> Tcm2/1
  Multiport Switch2/1 -> Tcm3/1
  Subtract3/1 -> Multiport Switch/5, Multiport Switch/6, Multiport Switch1/3, Multiport Switch1/7, Multiport Switch2/2, Multiport Switch2/4

== system EDS_Simulink_Model_02/Control Systetm 2 (FOC & SVPWM)/SVPWM 2/X.Y.Z 2 ==
  T : Inport
  Valpha : Inport  Port=2
  Vbeta : Inport  Port=3
  Vdc : Inport  Port=4
  Divide : Product  Inputs=**/
  Divide1 : Product  Inputs=**/
  Divide2 : Product  Inputs=**/
  Gain : Gain  Gain=sqrt(3)/3
  Gain1 : Gain  Gain=sqrt(3)
  Gain2 : Gain  Gain=1.5
  Gain3 : Gain  Gain=1.5
  Subtract : Sum
  Subtract1 : Sum  Inputs=+-
  X : Outport  VectorParamsAs1DForOutWhenUnconnected=off
  Y : Outport  Port=2  VectorParamsAs1DForOutWhenUnconnected=off
  Z : Outport  Port=3  VectorParamsAs1DForOutWhenUnconnected=off
  wires:
  Gain/1 -> Subtract1/1, Subtract/1
  Gain1/1 -> Divide/1
  T/1 -> Divide2/2, Divide1/2, Divide/2
  Vdc/1 -> Divide2/3, Divide1/3, Divide/3
  Valpha/1 -> Subtract1/2, Subtract/2
  Subtract/1 -> Divide1/1
  Subtract1/1 -> Divide2/1
  Divide/1 -> X/1
  Divide1/1 -> Gain2/1
  Divide2/1 -> Gain3/1
  Gain2/1 -> Y/1
  Gain3/1 -> Z/1
  Vbeta/1 -> Gain/1, Gain1/1

== system EDS_Simulink_Model_02/Control Systetm 2 (FOC & SVPWM)/SVPWM 2/produce PWM ==
  Tcm1 : Inport
  Tcm2 : Inport  Port=2
  Tcm3 : Inport  Port=3
  Bus Creator : BusCreator  Inputs=6
  Data Type Conversion : DataTypeConversion  OutDataTypeStr=double  SaturateOnIntegerOverflow=off  RndMeth=Floor
  Data Type Conversion1 : DataTypeConversion  OutDataTypeStr=double  SaturateOnIntegerOverflow=off  RndMeth=Floor
  Data Type Conversion2 : DataTypeConversion  OutDataTypeStr=double  SaturateOnIntegerOverflow=off  RndMeth=Floor
  Logical Operator : Logic  Operator=NOT  AllPortsSameDT=off
  Logical Operator1 : Logic  Operator=NOT  AllPortsSameDT=off
  Logical Operator2 : Logic  Operator=NOT  AllPortsSameDT=off
  Relay : Relay
  Relay1 : Relay
  Relay2 : Relay
  Sawtooth 2 : Subsystem
  Scope2 : Scope  NumInputPorts=4
  Subtract : Sum  Inputs=+-
  Subtract1 : Sum  Inputs=+-
  Subtract2 : Sum  Inputs=+-
  pulse : Outport  VectorParamsAs1DForOutWhenUnconnected=off
  wires:
  Subtract/1 -> Relay/1
  Subtract1/1 -> Relay1/1
  Subtract2/1 -> Relay2/1
  Logical Operator1/1 -> Data Type Conversion1/1
  Logical Operator2/1 -> Data Type Conversion2/1
  Logical Operator/1 -> Data Type Conversion/1
  Relay/1 -> Bus Creator/1, Logical Operator/1
  Relay1/1 -> Bus Creator/3, Logical Operator1/1
  Relay2/1 -> Bus Creator/5, Logical Operator2/1
  Bus Creator/1 -> pulse/1
  Data Type Conversion/1 -> Bus Creator/2
  Data Type Conversion1/1 -> Bus Creator/4
  Data Type Conversion2/1 -> Bus Creator/6
  Tcm1/1 -> Scope2/2, Subtract/2
  Sawtooth 2/1(pulses) -> Scope2/1, Subtract/1, Subtract2/1, Subtract1/1
  Tcm3/1 -> Scope2/4, Subtract2/2
  Tcm2/1 -> Scope2/3, Subtract1/2

== system EDS_Simulink_Model_02/Control Systetm 1 (FOC & SVPWM)/SVPWM 1/PWM Generation 1/Carrier Wave Generator ==
  Integrator : Integrator
  Pulse Generator : DiscretePulseGenerator  PulseType=Time based  Period=0.0001  PulseWidth=50
  Sum1 : Sum  Inputs=-+|  InputSameDT=on  SaturateOnIntegerOverflow=on  OutDataTypeStr=Inherit: Same as first input
  modulation index2 : Gain  Gain=2  SaturateOnIntegerOverflow=on  OutDataTypeStr=Inherit: Same as input  ParamDataTypeStr=Inherit: Same as input
  pi/1 : Constant
  Carrier Wave : Outport  VectorParamsAs1DForOutWhenUnconnected=off
  wires:
  pi/1/1 -> Sum1/1
  modulation index2/1 -> Sum1/2
  Sum1/1 -> Integrator/1
  Integrator/1 -> Carrier Wave/1
  Pulse Generator/1 -> modulation index2/1

== system EDS_Simulink_Model_02/Control Systetm 2 (FOC & SVPWM)/SVPWM 2/produce PWM/Sawtooth 2 ==
  Integrator : Integrator
  Pulse Generator : DiscretePulseGenerator  PulseType=Time based  Period=0.0001  PulseWidth=50
  Sum1 : Sum  Inputs=-+|  InputSameDT=on  SaturateOnIntegerOverflow=on  OutDataTypeStr=Inherit: Same as first input
  modulation index2 : Gain  Gain=2  SaturateOnIntegerOverflow=on  OutDataTypeStr=Inherit: Same as input  ParamDataTypeStr=Inherit: Same as input
  pi/1 : Constant
  pulses : Outport  VectorParamsAs1DForOutWhenUnconnected=off
  wires:
  pi/1/1 -> Sum1/1
  modulation index2/1 -> Sum1/2
  Sum1/1 -> Integrator/1
  Integrator/1 -> pulses/1
  Pulse Generator/1 -> modulation index2/1

== matlab function EDS_Simulink_Model_02/Electronic Differential System (EDS)/difference speed Δω calculation ==
  data: delta input; wv input; dw output; d parameter; L parameter; pi parameter
function dw = dw_fun(delta, wv, d, L, pi)

% delta : input     : [deg] steering angle
% wv    : input     : [rad/s] vehicle angular speed according to the center of turn
% L     : parameter : [m] wheelbase or distance between two wheels and axes
% d     : parameter : [m] distance between the wheels of the same axle
% dw    : output    : [rad/s] the difference between wheel drive angular speeds

delta = delta * pi/180;          % convert steering angle delta from deg to rad
dw    = - d * tan(delta)/L * wv;

== matlab function EDS_Simulink_Model_02/Subsystem Gearbox - Wheel 1 (Left)/Gearbox 1 ==
  data: m_speed_1 input; w_speed_1 output; i_gear parameter
function w_speed_1  = Gear_fun_1(m_speed_1,i_gear)

% w : wheel
% m : motor
w_speed_1  = m_speed_1 / i_gear;



% function [w_speed_1, w_torque_1] = Gear_fun_1(m_speed_1,m_torque_1,i_gear,n_eff_gear)
% 
% % w : wheel
% % m : motor
% 
% w_torque_1 = m_torque_1 * i_gear * n_eff_gear;
% w_speed_1  = m_speed_1 / i_gear;

== matlab function EDS_Simulink_Model_02/Subsystem Gearbox - Wheel 2 (Right)/Gearbox 2 ==
  data: m_speed_2 input; w_speed_2 output; i_gear parameter
function w_speed_2  = Gear_fun_2(m_speed_2,i_gear)

% w : wheel
% m : motor
w_speed_2  = m_speed_2 / i_gear;

== matlab function EDS_Simulink_Model_02/Subsystem Gearbox - Wheel 1 (Left)/Wheel Torque Calculation 1 ==
  data: w1 input; Tw1 output; a parameter; fr parameter; Rw parameter; Cx parameter; S parameter; M parameter; density parameter; K_tor_all_1 parameter; g parameter
function Tw1 = Tw1_fun(w1, a, fr, Rw, Cx, S, M, density, K_tor_all_1, g)

% w1          : input     : [rad/s]  Angular speed of drive wheel 1 (left)
% a           : parameter : [deg]    Grade angle of the road
% fr          : parameter : [-]      Vehicle friction coefficient
% Rw          : parameter : [m]      Wheel radius
% M           : parameter : [kg]     Vehicle mass
% S           : parameter : [m^2]    Vehicle frontal area
% density     : parameter : [kg/m^3] Air density
% Cx          : parameter : [-]      Aerodynamic drag coefficient
% g           : parameter : [m/s^2]  Gravitational acceleration 
% K_tor_all_1 : parameter : [-]      Torque allocation in wheel 1
% Tslope      : parameter : [Nm]     Vehicle torque
% Ttire       : parameter : [Nm]     Tire torque
% Taero       : parameter : [Nm]     Aerodynamique torque
% Tw1         : output    : [Nm]     Load torque that wheel 1 have to overcome

Tslope = M*g*sin(a)*Rw;                
Ttire  = M*g*fr*Rw;                       
Taero  = 1/2*density*S*Cx*Rw^3*w1^2;        
Tw1    = K_tor_all_1* (Tslope + Ttire + Taero);

== matlab function EDS_Simulink_Model_02/Subsystem Gearbox - Wheel 2 (Right)/Wheel Torque Calculation 2 ==
  data: w2 input; Tw2 output; a parameter; fr parameter; Rw parameter; Cx parameter; S parameter; M parameter; density parameter; K_tor_all_2 parameter; g parameter
function Tw2 = Tw2_fun(w2, a, fr, Rw, Cx, S, M, density, K_tor_all_2, g)

% w2          : input     : [rad/s]  Angular speed of drive wheel 1 (left)
% a           : parameter : [deg]    Grade angle of the road
% fr          : parameter : [-]      Vehicle friction coefficient
% Rw          : parameter : [m]      Wheel radius
% M           : parameter : [kg]     Vehicle mass
% S           : parameter : [m^2]    Vehicle frontal area
% density     : parameter : [kg/m^3] Air density
% Cx          : parameter : [-]      Aerodynamic drag coefficient
% g           : parameter : [m/s^2]  Gravitational acceleration 
% K_tor_all_2 : parameter : [-]      Torque allocation in wheel 1
% Tslope      : parameter : [Nm]     Vehicle torque
% Ttire       : parameter : [Nm]     Tire torque
% Taero       : parameter : [Nm]     Aerodynamique torque
% Tw2         : output    : [Nm]     Load torque that wheel 1 have to overcome

Tslope = M*g*sin(a)*Rw;                
Ttire  = M*g*fr*Rw;                       
Taero  = 1/2*density*S*Cx*Rw^3*w2^2;        
Tw2    = K_tor_all_2* (Tslope + Ttire + Taero);

== matlab function EDS_Simulink_Model_02/Pedal/If Action Subsystem/fun3 ==
  data: x input; y output; accel parameter
function y = accel1_fun(x,accel)

y = accel*x;

== matlab function EDS_Simulink_Model_02/Pedal/If Action Subsystem1/fun3 ==
  data: y output; accel parameter; accel_time parameter
function y = accel1_fun(accel, accel_time)

y = accel*accel_time;

== matlab function EDS_Simulink_Model_02/Control Systetm 2 (FOC & SVPWM)/Clark Transformation 2/MATLAB Function ==
  data: u input; y output
function y = fcn(u)

y = (u(1)-0.5*(u(2)+u(3))) * sqrt(2/3);

== matlab function EDS_Simulink_Model_02/Control Systetm 2 (FOC & SVPWM)/Clark Transformation 2/MATLAB Function1 ==
  data: u input; y output
function y = fcn(u)

y = sqrt(3)/2*(u(2)-u(3)) * sqrt(2/3);

== matlab function EDS_Simulink_Model_02/Electronic Differential System (EDS)/center of turn angular speed ωv calculation ==
  data: w1_est input; w2_est input; wv output
function wv = wv_fun(w1_est, w2_est)

% w1_est : input : [rad/s] actual angular speed of drive wheel 1 (left)
% w2_est : input : [rad/s] actual angular speed of drive wheel 2 (right)
% wv     : outpt : [rad/s] vehicle angular speed according to the center of turn

wv = (w1_est + w2_est) / 2;

== matlab function EDS_Simulink_Model_02/Reference Torque Calculation 1/Load Wheel Torque Calculation 1 ==
  data: w1 input; Tw1 output; a parameter; fr parameter; Rw parameter; Cx parameter; S parameter; M parameter; density parameter; K_tor_all_1 parameter; g parameter
function Tw1 = Tw1_fun(w1, a, fr, Rw, Cx, S, M, density, K_tor_all_1, g)

% w1          : input     : [rad/s]  Angular speed of drive wheel 1 (left)
% a           : parameter : [deg]    Grade angle of the road
% fr          : parameter : [-]      Vehicle friction coefficient
% Rw          : parameter : [m]      Wheel radius
% M           : parameter : [kg]     Vehicle mass
% S           : parameter : [m^2]    Vehicle frontal area
% density     : parameter : [kg/m^3] Air density
% Cx          : parameter : [-]      Aerodynamic drag coefficient
% g           : parameter : [m/s^2]  Gravitational acceleration 
% K_tor_all_1 : parameter : [-]      Torque allocation in wheel 1
% Tslope      : parameter : [Nm]     Vehicle torque
% Ttire       : parameter : [Nm]     Tire torque
% Taero       : parameter : [Nm]     Aerodynamique torque
% Tw1         : output    : [Nm]     Load torque that wheel 1 have to overcome

Tslope = M*g*sin(a)*Rw;                
Ttire  = M*g*fr*Rw;                       
Taero  = 1/2*density*S*Cx*Rw^3*w1^2;        
Tw1    = K_tor_all_1* (Tslope + Ttire + Taero);

== matlab function EDS_Simulink_Model_02/Reference Torque Calculation 2/Load Wheel Torque Calculation 2 ==
  data: w2 input; Tw2 output; a parameter; fr parameter; Rw parameter; Cx parameter; S parameter; M parameter; density parameter; K_tor_all_2 parameter; g parameter
function Tw2  = Tw2_fun(w2, a, fr, Rw, Cx, S, M, density, K_tor_all_2, g)

% w2          : input     : [rad/s]  Angular speed of drive wheel 2 (right)
% a           : parameter : [deg]    Grade angle of the road
% fr          : parameter : [-]      Vehicle friction coefficient
% Rw          : parameter : [m]      Wheel radius
% M           : parameter : [kg]     Vehicle mass
% S           : parameter : [m^2]    Vehicle frontal area
% density     : parameter : [kg/m^3] Air density
% Cx          : parameter : [-]      Aerodynamic drag coefficient
% g           : parameter : [m/s^2]  Gravitational acceleration 
% K_tor_all_2 : parameter : [-]      Torque allocation in wheel 2
% Tslope      : parameter : [Nm]     Vehicle torque
% Ttire       : parameter : [Nm]     Tire torque
% Taero       : parameter : [Nm]     Aerodynamique torque
% Tw2         : output    : [Nm]     Load torque that wheel 2 have to overcome

Tslope = M*g*sin(a)*Rw;                 
Ttire  = M*g*fr*Rw;                      
Taero  = 1/2*density*S*Cx*Rw^3*w2^2;     
Tw2    = K_tor_all_2 * (Tslope + Ttire + Taero);
